simulink model "Problem13_model_v2"  (R2020b)
settings: Solver=ode4  StartTime=0.0  StopTime=SIM_TIME  FixedStep=STEP_SIZE  RelTol=1e-3
values from neighbouring files (symbols this model uses):
  feff = 2.4*10^(-5)    (= 2.4e-05)    [problem12.m]    (also in problem13.m; problem15.m; problem16.m; problem17.m)
  Jeff = 1/n^2 .* supD + J_M    [Problem7_9.m]    (also in problem12.m = [0.0188, 0.0188, 0.0027, 0.0004].'; problem13.m = [0.0188, 0.0188, 0.0027, 0.0004].'; problem15.m = [0.0188, 0.0188, 0.0027, 0.0004].'; problem16.m = [0.0188, 0.0188, 0.0027, 0.0004].')
  K_D = 2*zeta/omega_n * K_p - feff / kT    [problem12.m]    (also in problem13.m; problem15.m = (2*omega_n*zeta*tau_i + 1 - feff) ./ kT; problem16.m = (2*omega_n*zeta*tau_i + 1 - feff) ./ kT; problem17.m = (2*omega_n*zeta*tau_i + 1 - feff) ./ kT)
  K_p = omega_n^2 * Jeff / kT    [problem12.m]    (also in problem13.m; problem15.m = (omega_n.^2*tau_i + 2*omega_n*zeta) ./ kT; problem16.m = (omega_n.^2*tau_i + 2*omega_n*zeta) ./ kT; problem17.m = (omega_n.^2*tau_i + 2*omega_n*zeta) ./ kT)
  kT = 0.17    [problem12.m]    (also in problem13.m; problem15.m; problem16.m; problem17.m)
  n = 53    [Problem7_9.m]    (also in Problem8_script.m = length(t); problem12.m; problem13.m; problem15.m)
  qr = [0.34, 0.34, 0.34, 0.34]    [problem12.m]    (also in problem13.m = [0.35, 0.35, 0.35, 0.35]; problem15.m = [0.35, 0.35, 0.35, 0.35]; problem16.m = [0.35, 0.35, 0.35, 0.35]; problem17.m = simout.qr)
  STEP_SIZE = 0.1    [Problem8_script.m]    (also in problem12.m = 0.01; problem13.m = 0.01; problem15.m = 0.001; problem16.m = 0.001)
  T_L = h    [problem13.m]    (also in problem15.m = zeros(4,1); problem16.m = zeros(4,1); problem17.m = abs(h); problem18.m = abs(h))
settings Model: Creator=Theis  LastModifiedBy=Theis

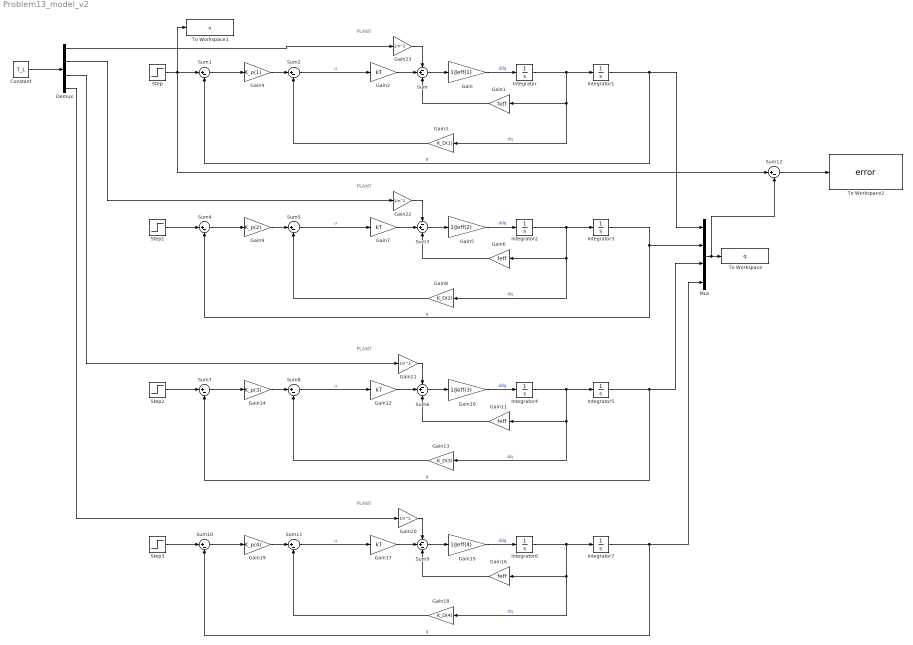
== system Problem13_model_v2 ==
  note: PLANT
  note: PLANT
  note: PLANT
  note: PLANT
  Constant : Constant  Value=T_L
  Demux : Demux
  Gain : Gain  Gain=1/Jeff(1)
  Gain{1,6,11,16} (4 alike) : Gain  Gain=feff
  Gain10 : Gain  Gain=1/Jeff(3)
  Gain{2,7,12,17} (4 alike) : Gain  Gain=kT
  Gain13 : Gain  Gain=K_D(3)
  Gain14 : Gain  Gain=K_p(3)
  Gain15 : Gain  Gain=1/Jeff(4)
  Gain18 : Gain  Gain=K_D(4)
  Gain19 : Gain  Gain=K_p(4)
  Gain{20..23} (4 alike) : Gain  Gain=1/n^2
  Gain3 : Gain  Gain=K_D(1)
  Gain4 : Gain  Gain=K_p(1)
  Gain5 : Gain  Gain=1/Jeff(2)
  Gain8 : Gain  Gain=K_D(2)
  Gain9 : Gain  Gain=K_p(2)
  Integrator{,1..7} (8 alike) : Integrator
  Mux : Mux
  Step{,1..3} (4 alike) : Step  Time=STEP_SIZE  After=qr(1)  SampleTime=0
  Sum{,3,6,9} (4 alike) : Sum  Inputs=-+-
  Sum{1..2,4..5,7..8,10..12} (9 alike) : Sum  Inputs=|+-
  To Workspace : ToWorkspace  VariableName=q  SaveFormat=Timeseries  SampleTime=-1
  To Workspace1 : ToWorkspace  VariableName=u  SaveFormat=Timeseries  SampleTime=-1
  To Workspace2 : ToWorkspace  VariableName=error  SaveFormat=Timeseries  SampleTime=-1
  wires:
  Integrator/1 -> Integrator1/1, Gain3/1, Gain1/1  "dq"
  Gain/1 -> Integrator/1  "ddq"
  Sum/1 -> Gain/1
  Sum2/1 -> Gain2/1  "u"
  Step/1 -> Sum12/1, To Workspace1/1, Sum1/1
  Integrator1/1 -> Mux/1, Sum1/2  "q"
  Gain3/1 -> Sum2/2
  Sum1/1 -> Gain4/1
  Gain4/1 -> Sum2/1
  Step1/1 -> Sum4/1
  Gain6/1 -> Sum3/3
  Gain7/1 -> Sum3/2
  Gain8/1 -> Sum5/2
  Gain9/1 -> Sum5/1
  Sum5/1 -> Gain7/1  "u"
  Sum3/1 -> Gain5/1
  Gain5/1 -> Integrator2/1  "ddq"
  Integrator2/1 -> Integrator3/1, Gain8/1, Gain6/1  "dq"
  Sum4/1 -> Gain9/1
  Integrator3/1 -> Mux/2, Sum4/2  "q"
  Gain13/1 -> Sum8/2
  Sum8/1 -> Gain12/1  "u"
  Sum6/1 -> Gain10/1
  Integrator4/1 -> Integrator5/1, Gain13/1, Gain11/1  "dq"
  Gain10/1 -> Integrator4/1  "ddq"
  Integrator7/1 -> Mux/4, Sum10/2  "q"
  Gain14/1 -> Sum8/1
  Sum10/1 -> Gain19/1
  Gain12/1 -> Sum6/2
  Integrator6/1 -> Integrator7/1, Gain18/1, Gain16/1  "dq"
  Sum9/1 -> Gain15/1
  Gain15/1 -> Integrator6/1  "ddq"
  Gain18/1 -> Sum11/2
  Step2/1 -> Sum7/1
  Step3/1 -> Sum10/1
  Sum11/1 -> Gain17/1  "u"
  Integrator5/1 -> Mux/3, Sum7/2  "q"
  Gain17/1 -> Sum9/2
  Gain16/1 -> Sum9/3
  Sum7/1 -> Gain14/1
  Gain19/1 -> Sum11/1
  Gain11/1 -> Sum6/3
  Mux/1 -> Sum12/2, To Workspace/1
  Gain1/1 -> Sum/3
  Gain2/1 -> Sum/2
  Gain20/1 -> Sum9/1
  Gain21/1 -> Sum6/1
  Gain22/1 -> Sum3/1
  Gain23/1 -> Sum/1
  Constant/1 -> Demux/1
  Demux/1 -> Gain23/1
  Demux/2 -> Gain22/1
  Demux/3 -> Gain21/1
  Demux/4 -> Gain20/1
  Sum12/1 -> To Workspace2/1
